simulink model "ColorObjectTracking"  (R2025b)
settings: Solver=FixedStepDiscrete  StartTime=0.0  StopTime=inf  FixedStep=0.1  RelTol=1e-3
InitFcn:
  | if(~exist('RGB_image')) RGB_image = imread('peppers.png'); end
undefined symbols (not defined in the file): strel
libraries: simulink x4, visionsinks x2, visiontextngfix x2, visionstatistics x1, visionmorphops x1, dspstat3 x1, dspvision x1
settings Model: SimulationMode=accelerator  Creator=Bender  LastModifiedBy=Bender

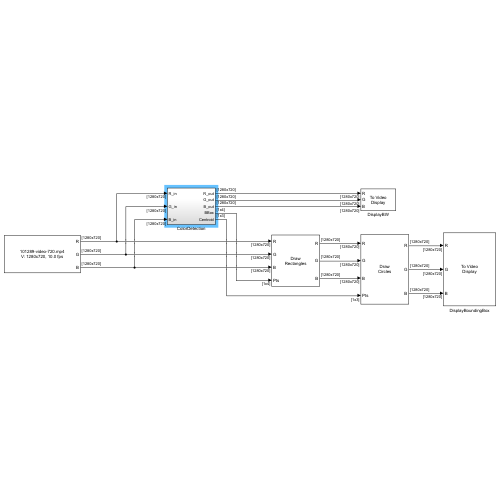
[thumbnail: Simulink's stored preview of the top-level diagram]
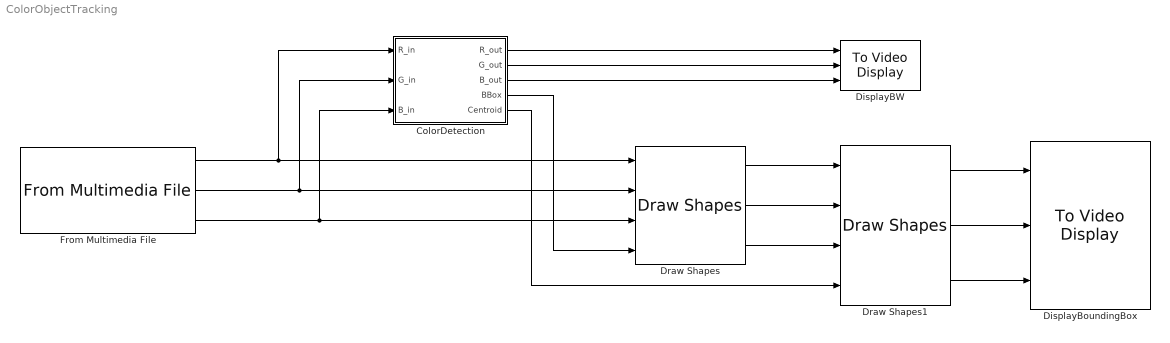
== system ColorObjectTracking ==
  ColorDetection : Subsystem
  DisplayBW : visionsinks/To Video Display  windowSizeMode=Normal  openAtMdlStart=on  fullScreen=off  videoWindowX=2  videoWindowY=45  saveWindowSize=off  videoWindowWidth=1196  videoWindowHeight=1481  inputColorFormat=RGB  inputType=Obsolete  imagePorts=Separate color signals  OutputDevice=On-screen video monitor  dataOrg=Column-major  isWindowOpen=off
  DisplayBoundingBox : visionsinks/To Video Display  windowSizeMode=Normal  openAtMdlStart=on  fullScreen=off  videoWindowX=1202  videoWindowY=45  saveWindowSize=off  videoWindowWidth=1196  videoWindowHeight=1481  inputColorFormat=RGB  inputType=Obsolete  imagePorts=Separate color signals  OutputDevice=On-screen video monitor  dataOrg=Column-major  isWindowOpen=off
  Draw Shapes : visiontextngfix/Draw Shapes  shape=Rectangles  fill=off  lineWidth=3  fillClrSource=Specify via dialog  display=White  intensity=200  color=[200 255 100]  opacity=0.6  viewport=Entire image  antialiasing=off  inType=Obsolete  imagePorts=Separate color signals  roundingMode=Floor  overflowMode=off  memoryMode=Specify word length  memoryWordLength=16  prodOutputMode=Binary point scaling  prodOutputWordLength=32  prodOutputFracLength=14  memoryFracLength=15
  Draw Shapes1 : visiontextngfix/Draw Shapes  shape=Circles  fill=on  lineWidth=3  fillClrSource=Specify via dialog  display=Black  intensity=200  color=[200 255 100]  opacity=0.6  viewport=Entire image  antialiasing=off  inType=Obsolete  imagePorts=Separate color signals  roundingMode=Floor  overflowMode=off  memoryMode=Specify word length  memoryWordLength=16  prodOutputMode=Binary point scaling  prodOutputWordLength=32  prodOutputFracLength=14  memoryFracLength=15
  From Multimedia File : dspvision/From Multimedia File  inputFilename=C:\Users\Bender\NextcloudFB\FB_DHBW\Robotik\Uebungen\Uebung3_Mobile_Roboter\4_ColorObjectTracking\101289-video-720.mp4  readRange=[1 Inf]  loop=on  numPlays=1  outputStreams=Video only  videoDataType=single  audioDataType=int16  inheritSampleTime=off  userDefinedSampleTime=0.1  noAudioOutput=off  isIntensityVideo=off  fourcc=RGB  colorVideoFormat=Separate color signals  outputEOF=off  dataOrg=Column-major  audioFrameSize=1024  computeAudioFrameSize=off  outSamplingMode=Sample based
      settings: LibrarySourceBlock=visionsources/From Multimedia File
  wires:
  From Multimedia File/1 -> Draw Shapes/1, ColorDetection/1(R_in)
  From Multimedia File/2 -> Draw Shapes/2, ColorDetection/2(G_in)
  From Multimedia File/3 -> Draw Shapes/3, ColorDetection/3(B_in)
  ColorDetection/1(R_out) -> DisplayBW/1
  ColorDetection/2(G_out) -> DisplayBW/2
  ColorDetection/3(B_out) -> DisplayBW/3
  ColorDetection/4(BBox) -> Draw Shapes/4
  Draw Shapes/1 -> Draw Shapes1/1
  Draw Shapes/2 -> Draw Shapes1/2
  Draw Shapes/3 -> Draw Shapes1/3
  ColorDetection/5(Centroid) -> Draw Shapes1/4
  Draw Shapes1/1 -> DisplayBoundingBox/1
  Draw Shapes1/2 -> DisplayBoundingBox/2
  Draw Shapes1/3 -> DisplayBoundingBox/3

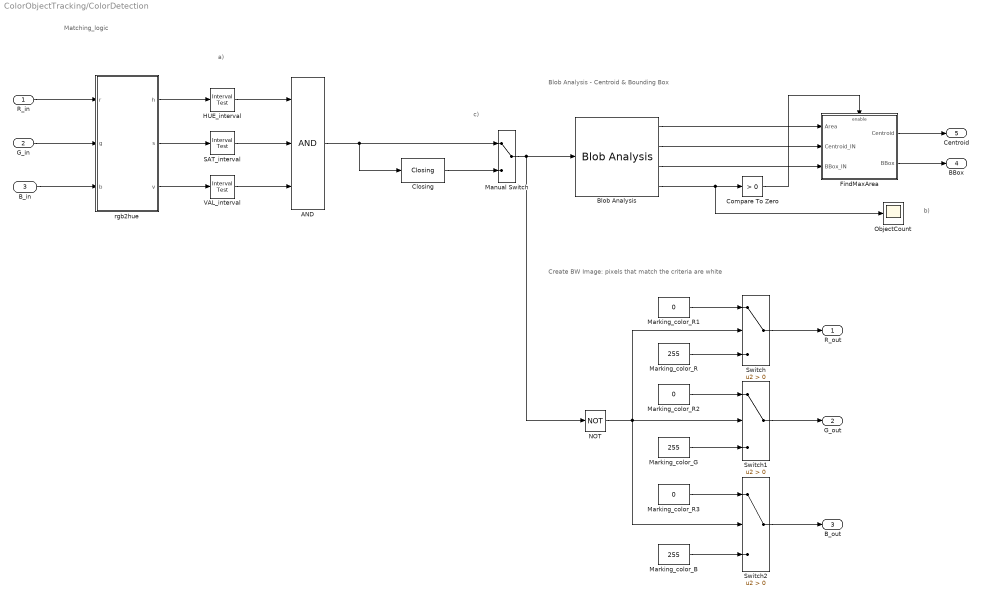
== system ColorObjectTracking/ColorDetection ==
  note: a)
  note: Create BW Image: pixels that match the criteria are white
  note: Blob Analysis - Centroid & Bounding Box
  note: Matching_logic
  note: b)
  note: c)
  R_in : Inport
  G_in : Inport  Port=2
  B_in : Inport  Port=3
  AND : Logic  Inputs=3  AllPortsSameDT=off  OutDataTypeStr=boolean
  Blob Analysis : visionstatistics/Blob Analysis  Tag=vipblks_row_conv  area=on  centroid=on  bBox=on  majorAxis=off  minorAxis=off  angle=off  eccentricity=off  equivDiameterSq=off  extent=off  perimeter=off  outDT=double  conn=8  isLabel=off  maxBlobs=50  warnIfNumBlobsExceeded=on  isCount=on  useMinArea=on  minArea=3000  useMaxArea=off  maxArea=intmax('uint32')  excludeBorderBlob=off  isOutVarDim=off  isFill=on  fillValues=-1  roundingMode=Floor  overflowMode=off  prodOutputMode=Binary point scaling  prodOutputWordLength=32  prodOutputFracLength=16  accumMode=Binary point scaling  accumWordLength=32  accumFracLength=0  outputMode=Binary point scaling  outputWordLength=32  outputFracLength=16  firstCoeffMode=Binary point scaling  firstCoeffWordLength=16  firstCoeffFracLength=14  secondCoeffMode=Binary point scaling  secondCoeffWordLength=32  secondCoeffFracLength=16
  Closing : visionmorphops/Closing  nhoodsrc=Specify via dialog  strel=strel('line',15,45)
  Compare To Zero : simulink/Logic and Bit Operations/Compare To Zero  relop=>  OutDataTypeStr=boolean
  FindMaxArea : Subsystem  TreatAsAtomicUnit=on
  HUE_interval : simulink/Logic and Bit Operations/Interval Test  IntervalClosedRight=on  uplimit=1  IntervalClosedLeft=on  lowlimit=0  OutDataTypeStr=boolean
  Manual Switch : ManualSwitch
  Marking_color_B : Constant  Value=255
  Marking_color_G : Constant  Value=255
  Marking_color_R : Constant  Value=255
  Marking_color_R1 : Constant  Value=0
  Marking_color_R2 : Constant  Value=0
  Marking_color_R3 : Constant  Value=0
  NOT : Logic  Operator=NOT  AllPortsSameDT=off  OutDataTypeStr=boolean
  ObjectCount : Scope
      settings: ActiveDisplayYMinimum=0.9  ActiveDisplayYMaximum=1.1
  SAT_interval : simulink/Logic and Bit Operations/Interval Test  IntervalClosedRight=on  uplimit=1  IntervalClosedLeft=on  lowlimit=0  OutDataTypeStr=boolean
  Switch : Switch  Criteria=u2 > Threshold  OutDataTypeStr=uint8  SaturateOnIntegerOverflow=off  InputSameDT=off
  Switch1 : Switch  Criteria=u2 > Threshold  OutDataTypeStr=uint8  SaturateOnIntegerOverflow=off  InputSameDT=off
  Switch2 : Switch  Criteria=u2 > Threshold  OutDataTypeStr=uint8  SaturateOnIntegerOverflow=off  InputSameDT=off
  VAL_interval : simulink/Logic and Bit Operations/Interval Test  IntervalClosedRight=on  uplimit=1  IntervalClosedLeft=on  lowlimit=0  OutDataTypeStr=boolean
  rgb2hue : MATLAB Function  TreatAsAtomicUnit=on
  R_out : Outport
  G_out : Outport  Port=2
  B_out : Outport  Port=3
  BBox : Outport  Port=4
  Centroid : Outport  Port=5
  wires:
  NOT/1 -> Switch2/2, Switch1/2, Switch/2
  rgb2hue/3(v) -> VAL_interval/1
  rgb2hue/1(h) -> HUE_interval/1
  G_in/1 -> rgb2hue/2(g)
  rgb2hue/2(s) -> SAT_interval/1
  B_in/1 -> rgb2hue/3(b)
  R_in/1 -> rgb2hue/1(r)
  Marking_color_R/1 -> Switch/3
  Switch/1 -> R_out/1
  Switch1/1 -> G_out/1
  Switch2/1 -> B_out/1
  Marking_color_G/1 -> Switch1/3
  Marking_color_B/1 -> Switch2/3
  HUE_interval/1 -> AND/1
  SAT_interval/1 -> AND/2
  VAL_interval/1 -> AND/3
  AND/1 -> Closing/1, Manual Switch/1
  Marking_color_R1/1 -> Switch/1
  Marking_color_R2/1 -> Switch1/1
  Marking_color_R3/1 -> Switch2/1
  Manual Switch/1 -> NOT/1, Blob Analysis/1
  Closing/1 -> Manual Switch/2
  Blob Analysis/4 -> ObjectCount/1, Compare To Zero/1
  Compare To Zero/1 -> FindMaxArea/Enable
  Blob Analysis/1 -> FindMaxArea/1(Area)
  Blob Analysis/2 -> FindMaxArea/2(Centroid_IN)
  Blob Analysis/3 -> FindMaxArea/3(BBox_IN)
  FindMaxArea/1(Centroid) -> Centroid/1
  FindMaxArea/2(BBox) -> BBox/1

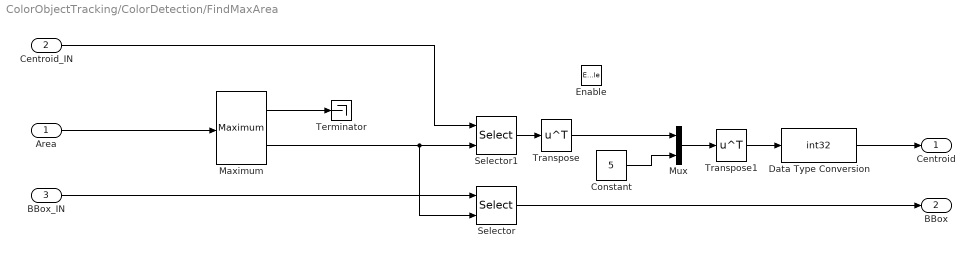
== system ColorObjectTracking/ColorDetection/FindMaxArea ==
  Area : Inport
  Centroid_IN : Inport  Port=2
  BBox_IN : Inport  Port=3
  Enable : EnablePort
  Constant : Constant  Value=5
  Data Type Conversion : DataTypeConversion  OutDataTypeStr=int32  SaturateOnIntegerOverflow=off  RndMeth=Floor
  Maximum : dspstat3/Maximum  operation=maximum  fcn=Value and Index  indexBase=One  operateOver=Each column  Dimension=1  InputProcessing=Columns as channels (frame based)  reset=None  roiEnable=off  roiType=Rectangles  roiPortion=Entire ROI  roiOutput=Individual statistics for each ROI  roiFlag=off  roundingMode=Floor  overflowMode=off  accumDataTypeStr=Inherit: Same as product output  accumLastDataTypeStr=Inherit: Same as product output
      settings: LibrarySourceBlock=dsphdlsupportstat/Maximum
  Mux : Mux  Inputs=2
  Selector : Selector  NumberOfDimensions=2  InputPortWidth=3  IndexOptions=Index vector (port),Select all  Indices=[1],1  OutputSizes=1,1
  Selector1 : Selector  NumberOfDimensions=2  InputPortWidth=3  IndexOptions=Index vector (port),Select all  Indices=[1],1  OutputSizes=1,1
  Terminator : Terminator
  Transpose : Math  Operator=transpose
  Transpose1 : Math  Operator=transpose
  Centroid : Outport
  BBox : Outport  Port=2
  wires:
  Centroid_IN/1 -> Selector1/1
  Selector/1 -> BBox/1
  Data Type Conversion/1 -> Centroid/1
  Transpose/1 -> Mux/1
  Maximum/2 -> Selector/2, Selector1/2
  Transpose1/1 -> Data Type Conversion/1
  Selector1/1 -> Transpose/1
  Mux/1 -> Transpose1/1
  BBox_IN/1 -> Selector/1
  Constant/1 -> Mux/2
  Area/1 -> Maximum/1
  Maximum/1 -> Terminator/1

== matlab function ColorObjectTracking/ColorDetection/rgb2hue ==
  data: r input; h output; g input; b input; s output; v output
function [h,s,v] = rgb2hue(r,g,b)
%#codegen

sz = size(r);
r_re = double(reshape(r,[sz(1)*sz(2),1]))/255.0;
g_re = double(reshape(g,[sz(1)*sz(2),1]))/255.0;
b_re = double(reshape(b,[sz(1)*sz(2),1]))/255.0;
hsv = rgb2hsv([r_re,g_re,b_re]);
h = reshape(hsv(:,1), sz);
s = reshape(hsv(:,2), sz);
v = reshape(hsv(:,3), sz);
